simulink model "vehicle_motion_model_final_temp"  (R2021b)
settings: Solver=ode5  StartTime=0.0  StopTime=600  FixedStep=0.001  RelTol=1e-3
StopFcn:
  | % stop simulation callback function
  | figure(1);
  | out.x_gt.data = permute(out.x_gt.data,[3, 1, 2]);
  | plot3(out.x_gt.data(:, 1), out.x_gt.data(:, 2), -out.x_gt.data(:, 3), 'Color', 'r', 'LineWidth', 1.5);
  | legend('Истинная траектория')
  | xlabel('X, \itм');
  | ylabel('Y, \itм');
  | zlabel('Z, \itм');
  | figure(2);
  | plot3(out.x.data(:, 1), out.x.data(:, 2), -out.x.data(:, 3), 'Color', 'b', 'LineWidth', 1.5);
  | hold on;
  | xlabel('X, \itм');
  | ylabel('Y, \itм');
  | zlabel('Z, \itм');
  | % legend('pos')
  | hold on;
  | plot3(out.x_gt.data(:, 1), out.x_gt.data(:, 2), -out.x_gt.data(:, 3), 'Color', 'r', 'LineWidth', 1.5);
  | hold on;
  | legend('Рассчитанная траектория', 'Истинная траектория')
  | % errors
  | figure(3);
  | yyaxis left;
  | plot(out.hor_err_fus.time, out.hor_err_fus.data, 'Color', 'b', 'LineWidth', 1.5);
  | xlabel('время, \itс');
  | ylabel('Горизонтальная ошибка, \itм');
  | hold on;
  | yyaxis right;
  | plot(out.ver_err_fus.time, out.ver_err_fus.data, 'Color', 'r', 'LineWidth', 1.5);
  | ylabel('Вертикальная ошибка, \itм');
  | legend('Горизонтальная позиционная ошибка', 'Вертикальная позиционная ошибка');
  | grid on;
  | figure(4);
  | yyaxis left;
  | plot(out.hor_err_ins.time, out.hor_err_ins.data, '-', 'Color', 'b', 'LineWidth', 1.5);
  | xlabel('время, \itс');
  | ylabel('Горизонтальная ошибка, \itм');
  | hold on;
  | yyaxis right;
  | plot(out.ver_err_ins.time, out.ver_err_ins.data, '-', 'Color', 'r', 'LineWidth', 1.5);
  | ylabel('Вертикальная ошибка, \itм');
  | legend('Горизонтальная позиционная ошибка', 'Вертикальная позиционная ошибка');
  | grid on;
model workspace (MAT data in the model file):
  AxlIxx = 62.3745166667
  AxlM = 160
  Cps = 2
  CzWhlAxl = 557955.087061
  DCT_Param : object (value not decoded)
  Downshift_Speeds = [9.5625 12.9375 16.3125 19.6875 23.0625 26.4375 29.8125 33.1875 36.5625 39.9375 43.3125 46.6875 ... (28 elements, 4x7)]
  F0zWhlAxl = 16132.2380068
  HTCH : object (value not decoded)
  Hmax = 0.25
  KzWhlAxl = 58428920.0848
  NCyl = 6
  Pedal_Positions = [0.1 0.4 0.5 0.9]
  Pstd = 101325
  Q = [1  0  0; 0  1  0; 0  0  1]
  Rair = 287
  SUS : object (value not decoded)
  TRA : object (value not decoded)
  Trans : object (value not decoded)
  Tstd = 293.15
  Upshift_Speeds = [12.9375 16.3125 19.6875 33 26.4375 29.8125 33.1875 52.5 39.9375 43.3125 46.6875 77.25 ... (28 elements, 4x7)]
  VEH : object (value not decoded)
  Vd = 0.00346
  WH : Mass (value not decoded)
  dt3D = 0.05
  f_air = [0 0 0 0 0 0 0 0 0 0 0 0 ... (256 elements, 16x16)]
  f_co = [0 0 0 0 0 0 0 0 0 0 0 0 ... (256 elements, 16x16)]
  f_co2 = [0 0 0 0 0 0 0 0 0 0 0 0 ... (256 elements, 16x16)]
  f_eff = [352.135682859 352.135682859 320.724378192 303.655312657 295.930136708 291.240087194 291.240271258 291.240312459 291.240275452 291.240198499 291.240100781 291.240018769 ... (256 elements, 16x16)]
  f_fuel = [0 0 0 0 0 0 0 0 0 0 0 0 ... (256 elements, 16x16)]
  f_hc = [0 0 0 0 0 0 0 0 0 0 0 0 ... (256 elements, 16x16)]
  f_nox = [0 0 0 0 0 0 0 0 0 0 0 0 ... (256 elements, 16x16)]
  f_pm = [0 0 0 0 0 0 0 0 0 0 0 0 ... (256 elements, 16x16)]
  f_susp_axl_bp = [1 2]
  f_susp_dz_bp = [-0.325022776267 -0.315022776267 -0.305022776267 -0.205022776267 -0.105022776267 -0.00502277626717 0.0949772237328 0.194977223733 0.204977223733 0.214977223733]
  f_susp_dzdot_bp = [-3 -0.3 -0.2 -0.1 0 0.1 0.2 0.3 3]
  f_susp_fmz = [-144070.391448 -93629.24037 -75929.1118915 -20630.5828179 -15385.48216 -10140.3815021 -4895.28084414 349.819813785 -31916.3973792 18437.6709544 -83996.1993354 -33555.0482577 ... (43920 elements, 10x9x61x2x4)]
  f_susp_geom = [0 0 0 0 0 0 0 0 0 0 0 0 ... (3660 elements, 10x61x2x3)]
  f_susp_strgdelta_bp = [-0.523598775598 -0.506145483078 -0.488692190558 -0.471238898038 -0.453785605519 -0.436332312999 -0.418879020479 -0.401425727959 -0.383972435439 -0.366519142919 -0.349065850399 -0.331612557879 ... (61 elements, 1x61)]
  f_tbrake = [0 76.8593923996 105.140482948 131.533638111 157.926793274 176.658631717 176.65727296 176.656856686 176.656879077 176.657093756 176.657404516 176.65772406 ... (256 elements, 16x16)]
  f_tbrake_n_bpt = [0 649.519052838 912.419621844 1175.32019085 1438.22075986 1701.12132886 1964.02189787 2226.92246687 2489.82303588 2752.72360489 3015.62417389 3278.5247429 ... (16 elements, 1x16)]
  f_tbrake_t_bpt = [0 34.6410161514 61.0341713143 87.4273264773 113.82048164 140.213636803 166.606791966 192.999947129 219.393102292 245.786257455 272.179412618 298.572567781 ... (16 elements, 1x16)]
  f_texh = [766.752464599 766.752464599 786.17542386 801.679939032 884.591982581 910.574397722 910.571871054 910.570774534 910.570601632 910.570821151 910.571247242 910.571639815 ... (256 elements, 16x16)]
  f_twc_eff_co = [0.17 0.25 0.45 0.99 0.99 0.99 0.99]
  f_twc_eff_hc = [0.21 0.375 0.75 0.98 0.98 0.98 0.98]
  f_twc_eff_lam = [0.909090909 0.944055944 0.979020979 1 1.013986014 1.048951049 1.083916084]
  f_twc_eff_nox = [0.98 0.98 0.98 0.97 0.05 0.02 0]
  h = 0.134
symbols that are objects in the model workspace (value not decoded): VEH
libraries: aerolibcommonsys x8, sharedtransform x8, sharedutil x7, autolibsharedcommon x7, autolibutils x4, vehdynlibtirecommon x3, dspstat3 x2, mspsensorlib x1, aerolibnav x1, shared6dof x1, autolibshared x1, vehdynlibsuspension x1
(part 2 of 9)

== system vehicle_motion_model_final_temp/Axle Torque ==
  Vehicle : Inport
  1-D Lookup Table : Lookup_n-D  NumberOfTableDimensions=1  BreakpointsForDimension1=[0 3]  Table=[1 0.2]  InternalRulePriority=Speed  RndMeth=Simplest  InputSameDT=on
  1200 Nm Per Rear Wheel : Constant  Value=1200
  Bus Selector : BusSelector  OutputSignals=Vehicle.BdyFrm.Cg.Vel.xdot
  Constant : Constant  Value=0
  Mux : Mux
  Product : Product
  Transfer Fcn : TransferFcn  Denominator=[0.2 1]
  Axle Torque : Outport
  wires:
  Constant/1 -> Mux/2, Mux/1
  1200 Nm Per Rear Wheel/1 -> Product/2
  Transfer Fcn/1 -> Mux/4, Mux/3
  Mux/1 -> Axle Torque/1
  Vehicle/1 -> Bus Selector/1
  Bus Selector/1 -> 1-D Lookup Table/1  "<xdot>"
  Product/1 -> Transfer Fcn/1
  1-D Lookup Table/1 -> Product/1

== system vehicle_motion_model_final_temp/BINS ==
  note: block with biases drift
  note: adis 16384
  note: there will be an assumption for sensor fusion: we consider that IMU acc-ters are identical, so them noises are white, uncorreletad and isotopic (sphere) and therefore mean and covariance matrix are invariant upon rotations (?)
  inputIMU : Inport
  Bus Creator : BusCreator  Inputs=2
  Bus Selector : BusSelector  OutputSignals=Vehicle.BdyFrm.Cg.Abe,Vehicle.BdyFrm.Cg.AngVel,Vehicle.BdyFrm.Cg.AngAcc,Vehicle.BdyFrm.Cg.DCM
  Display : Display
  IMU : mspsensorlib/IMU  Commented=on  DispRefFrame=NED  Temperature=25  MagneticFieldNED=[ 27.5550, -2.4169, -16.0849 ]  MagneticFieldENU=[ -2.4169, 27.5550, 16.0849 ]  SeedDouble=67  SimulateUsing=Interpreted execution  AccelParamsMeasurementRange=Inf  AccelParamsResolution=0  AccelParamsConstantBias=[ 0, 0, 0 ]  AccelParamsAxesMisalignment=[ 100, 0, 0; 0, 100, 0; 0, 0, 100 ]  AccelParamsNoiseDensity=[ 0, 0, 0 ]  AccelParamsBiasInstability=[ 0, 0, 0 ]  AccelParamsRandomWalk=[ 0, 0, 0 ]  AccelParamsTemperatureBias=[ 0, 0, 0 ]  AccelParamsTemperatureScaleFactor=[ 0, 0, 0 ]  GyroParamsMeasurementRange=Inf  GyroParamsResolution=0  GyroParamsConstantBias=[ 0, 0, 0 ]  GyroParamsAxesMisalignment=[ 100, 0, 0; 0, 100, 0; 0, 0, 100 ]  GyroParamsAccelerationBias=[ 0, 0, 0 ]  GyroParamsNoiseDensity=[ 0, 0, 0 ]  GyroParamsBiasInstability=[ 0, 0, 0 ]  GyroParamsRandomWalk=[ 0, 0, 0 ]  GyroParamsTemperatureBias=[ 0, 0, 0 ]  GyroParamsTemperatureScaleFactor=[ 0, 0, 0 ]  MagParamsMeasurementRange=Inf  MagParamsResolution=0  MagParamsConstantBias=[ 0, 0, 0 ]  MagParamsAxesMisalignment=[ 100, 0, 0; 0, 100, 0; 0, 0, 100 ]  MagParamsNoiseDensity=[ 0, 0, 0 ]  MagParamsBiasInstability=[ 0, 0, 0 ]  MagParamsRandomWalk=[ 0, 0, 0 ]  MagParamsTemperatureBias=[ 0, 0, 0 ]  MagParamsTemperatureScaleFactor=[ 0, 0, 0 ]
      settings: SourceProductBaseCode=TF,NV
  Product : Product  Multiplication=Matrix(*)
  RMS : dspstat3/RMS  run=off  directionMode=Each column  dimension=1  reset_popup=None
  RMS1 : dspstat3/RMS  run=off  directionMode=Each column  dimension=1  reset_popup=None
  Scope1 : Scope  NumInputPorts=2
  Scope3 : Scope  NumInputPorts=2
  Subsystem : Subsystem
  Subsystem1 : Subsystem
  Three-axis Inertial Measurement Unit1 : aerolibnav/Three-axis Inertial Measurement Unit  units=Metric (MKS)  imu=[0 0 0]  i_Ts=0  dtype_a=off  w_a=190  z_a=0.707  a_sf_cc=[1 0 0; 0 1 0; 0 0 1]  a_bias=[0, 0, 0]  a_sat="[-inf  -inf  -inf  inf inf inf]"  dtype_g=off  w_g=190  z_g=0.707  g_sf_cc=[1 0 0; 0 1 0; 0 0 1]  g_bias=[0, 0, 0]  g_sens=[0 0 0]  g_sat="[-inf  -inf  -inf  inf inf inf]"  i_rand=on  i_seeds=[23093 23094 23095 23096 23097 23098]  i_pow=[6e-8 6e-8 6e-8 7e-9 7e-9 7e-9]
  Three-axis Inertial Measurement Unit2 : Subsystem  Commented=on  AncestorBlock=aerolibnav/Three-axis Inertial Measurement Unit  mask(Three-axis Inertial Measurement Unit){units=Metric (MKS), imu=[0 0 0], i_Ts=0.001, dtype_a=off, w_a=190, z_a=0.707, a_sf_cc=[1 0 0; 0 1 0; 0 0 1], a_bias=[3e-4,-4e-4, 1e-4], a_sat=[-inf  -inf  -inf  inf inf inf], dtype_g=off, w_g=190, z_g=0.707, g_sf_cc=[1 0 0; 0 1 0; 0 0 1], g_bias=[-2e-4, 4e-4, -1e-4], g_sens=[0 0 0], g_sat=[-inf  -inf  -inf  inf inf inf], i_rand=on, i_seeds=[23093 23094 23095 23096 23097 23098], i_pow=[6e-8 6e-8 6e-8 2e-12 2e-12 2e-12]}
      mask prompts: units "aeroblks:aeroblknav:blockThreeaxisInertialMeasurementUnitParamUnits"; imu "aeroblks:aeroblknav:blockThreeaxisInertialMeasurementUnitParamIMUlocation"; i_Ts "aeroblks:aeroblknav:blockThreeaxisInertialMeasurementUnitParamUpdaterate"; dtype_a "aeroblks:aeroblknav:blockThreeaxisInertialMeasurementUnitParamSecondorderdynamicsforaccelerometer"; w_a "aeroblks:aeroblknav:blockThreeaxisInertialMeasurementUnitParamAccelerometernaturalfrequencyradsec"; z_a "aeroblks:aeroblknav:blockThreeaxisInertialMeasurementUnitParamAccelerometerdampingratio"; a_sf_cc "aeroblks:aeroblknav:blockThreeaxisInertialMeasurementUnitParamAccelerometerscalefactorandcrosscoupling"; a_bias "aeroblks:aeroblknav:blockThreeaxisInertialMeasurementUnitParamAccelerometermeasurementbias"; a_sat "aeroblks:aeroblknav:blockThreeaxisInertialMeasurementUnitParamAccelerometerupperandlowerlimits"; dtype_g "aeroblks:aeroblknav:blockThreeaxisInertialMeasurementUnitParamSecondorderdynamicsforgyro"; w_g "aeroblks:aeroblknav:blockThreeaxisInertialMeasurementUnitParamGyronaturalfrequencyradsec"; z_g "aeroblks:aeroblknav:blockThreeaxisInertialMeasurementUnitParamGyrodampingratio"; g_sf_cc "aeroblks:aeroblknav:blockThreeaxisInertialMeasurementUnitParamGyroscalefactorsandcrosscoupling"; g_bias "aeroblks:aeroblknav:blockThreeaxisInertialMeasurementUnitParamGyromeasurementbias"; g_sens "aeroblks:aeroblknav:blockThreeaxisInertialMeasurementUnitParamGsensitivebias"; g_sat "aeroblks:aeroblknav:blockThreeaxisInertialMeasurementUnitParamGyroupperandlowerlimits"; i_rand "aeroblks:aeroblknav:blockThreeaxisInertialMeasurementUnitParamNoiseon"; i_seeds "aeroblks:aeroblknav:blockThreeaxisInertialMeasurementUnitParamNoiseseeds"; i_pow "aeroblks:aeroblknav:blockThreeaxisInertialMeasurementUnitParamNoisepower"
      mask help: aeroblks:aeroblknav:blockThreeaxisInertialMeasurementUnitDesc
      mask init:
      | block = gcb;   
      | ports=aeroicon('aeroblkimu','icon');
      mask Help: eval('asbhelp');
      mask TypeOptions units: aeroblks:aeroblknav:blockThreeaxisInertialMeasurementUnitParamComboMetricMKS | aeroblks:aeroblknav:blockThreeaxisInertialMeasurementUnitParamComboEnglish
      mask Callback dtype_a: aeroicon('aeroblkimu')
      mask Callback dtype_g: aeroicon('aeroblkimu')
      mask Callback i_rand: aeroicon('aeroblkimu')
      mask DialogControl ParameterTabVar0 Prompt: Main
      mask DialogControl units Prompt: Units:
      mask DialogControl imu Prompt: IMU location:
      mask DialogControl i_Ts Prompt: Update rate:
      mask DialogControl ParameterTabVar01 Prompt: Accelerometer
      mask DialogControl dtype_a Prompt: Second-order dynamics for accelerometer
      mask DialogControl w_a Prompt: Accelerometer natural frequency (rad/sec):
      mask DialogControl z_a Prompt: Accelerometer damping ratio:
      mask DialogControl a_sf_cc Prompt: Accelerometer scale factor and cross-coupling:
      mask DialogControl a_bias Prompt: Accelerometer measurement bias:
      mask DialogControl a_sat Prompt: Accelerometer upper and lower limits:
      mask DialogControl ParameterTabVar012 Prompt: Gyroscope
      mask DialogControl dtype_g Prompt: Second-order dynamics for gyro
      mask DialogControl w_g Prompt: Gyro natural frequency (rad/sec):
      mask DialogControl z_g Prompt: Gyro damping ratio:
      mask DialogControl g_sf_cc Prompt: Gyro scale factors and cross-coupling:
      mask DialogControl g_bias Prompt: Gyro measurement bias:
      mask DialogControl g_sens Prompt: G-sensitive bias:
      mask DialogControl g_sat Prompt: Gyro upper and lower limits:
      mask DialogControl ParameterTabVar0123 Prompt: Noise
      mask DialogControl i_rand Prompt: Noise on
      mask DialogControl i_seeds Prompt: Noise seeds:
      mask DialogControl i_pow Prompt: Noise power:
      mask Display:
      | port_label(ports(1).type,ports(1).port,ports(1).txt,'texmode','on');
      | port_label(ports(2).type,ports(2).port,ports(2).txt,'texmode','on');
      | port_label(ports(3).type,ports(3).port,ports(3).txt,'texmode','on');
      | port_label(ports(4).type,ports(4).port,ports(4).txt,'texmode','on');
      | port_label(ports(5).type,ports(5).port,ports(5).txt,'texmode','on');
      | port_label(ports(6).type,ports(6).port,ports(6).txt,'texmode','on');
      | port_label(ports(7).type,ports(7).port,ports(7).txt,'texmode','on');
  Three-axis Inertial Measurement Unit4 : Subsystem  Commented=on  AncestorBlock=aerolibnav/Three-axis Inertial Measurement Unit  mask(Three-axis Inertial Measurement Unit){units=Metric (MKS), imu=[0 0 0], i_Ts=0.01, dtype_a=off, w_a=190, z_a=0.707, a_sf_cc=[1 0 0; 0 1 0; 0 0 1], a_bias=[3e-4,-4e-4, 1e-4], a_sat=[-inf  -inf  -inf  inf inf inf], dtype_g=off, w_g=190, z_g=0.707, g_sf_cc=[1 0 0; 0 1 0; 0 0 1], g_bias=[-2e-4, 4e-4, -1e-4], g_sens=[0 0 0], g_sat=[-inf  -inf  -inf  inf inf inf], i_rand=on, i_seeds=[23093 23094 23095 23096 23097 23098], i_pow=[7e-9 7e-9 7e-9 6e-8 6e-8 6e-8]}
      mask prompts: units "aeroblks:aeroblknav:blockThreeaxisInertialMeasurementUnitParamUnits"; imu "aeroblks:aeroblknav:blockThreeaxisInertialMeasurementUnitParamIMUlocation"; i_Ts "aeroblks:aeroblknav:blockThreeaxisInertialMeasurementUnitParamUpdaterate"; dtype_a "aeroblks:aeroblknav:blockThreeaxisInertialMeasurementUnitParamSecondorderdynamicsforaccelerometer"; w_a "aeroblks:aeroblknav:blockThreeaxisInertialMeasurementUnitParamAccelerometernaturalfrequencyradsec"; z_a "aeroblks:aeroblknav:blockThreeaxisInertialMeasurementUnitParamAccelerometerdampingratio"; a_sf_cc "aeroblks:aeroblknav:blockThreeaxisInertialMeasurementUnitParamAccelerometerscalefactorandcrosscoupling"; a_bias "aeroblks:aeroblknav:blockThreeaxisInertialMeasurementUnitParamAccelerometermeasurementbias"; a_sat "aeroblks:aeroblknav:blockThreeaxisInertialMeasurementUnitParamAccelerometerupperandlowerlimits"; dtype_g "aeroblks:aeroblknav:blockThreeaxisInertialMeasurementUnitParamSecondorderdynamicsforgyro"; w_g "aeroblks:aeroblknav:blockThreeaxisInertialMeasurementUnitParamGyronaturalfrequencyradsec"; z_g "aeroblks:aeroblknav:blockThreeaxisInertialMeasurementUnitParamGyrodampingratio"; g_sf_cc "aeroblks:aeroblknav:blockThreeaxisInertialMeasurementUnitParamGyroscalefactorsandcrosscoupling"; g_bias "aeroblks:aeroblknav:blockThreeaxisInertialMeasurementUnitParamGyromeasurementbias"; g_sens "aeroblks:aeroblknav:blockThreeaxisInertialMeasurementUnitParamGsensitivebias"; g_sat "aeroblks:aeroblknav:blockThreeaxisInertialMeasurementUnitParamGyroupperandlowerlimits"; i_rand "aeroblks:aeroblknav:blockThreeaxisInertialMeasurementUnitParamNoiseon"; i_seeds "aeroblks:aeroblknav:blockThreeaxisInertialMeasurementUnitParamNoiseseeds"; i_pow "aeroblks:aeroblknav:blockThreeaxisInertialMeasurementUnitParamNoisepower"
      mask help: aeroblks:aeroblknav:blockThreeaxisInertialMeasurementUnitDesc
      mask init:
      | block = gcb;   
      | ports=aeroicon('aeroblkimu','icon');
      mask Help: eval('asbhelp');
      mask TypeOptions units: aeroblks:aeroblknav:blockThreeaxisInertialMeasurementUnitParamComboMetricMKS | aeroblks:aeroblknav:blockThreeaxisInertialMeasurementUnitParamComboEnglish
      mask Callback dtype_a: aeroicon('aeroblkimu')
      mask Callback dtype_g: aeroicon('aeroblkimu')
      mask Callback i_rand: aeroicon('aeroblkimu')
      mask DialogControl ParameterTabVar0 Prompt: Main
      mask DialogControl units Prompt: Units:
      mask DialogControl imu Prompt: IMU location:
      mask DialogControl i_Ts Prompt: Update rate:
      mask DialogControl ParameterTabVar01 Prompt: Accelerometer
      mask DialogControl dtype_a Prompt: Second-order dynamics for accelerometer
      mask DialogControl w_a Prompt: Accelerometer natural frequency (rad/sec):
      mask DialogControl z_a Prompt: Accelerometer damping ratio:
      mask DialogControl a_sf_cc Prompt: Accelerometer scale factor and cross-coupling:
      mask DialogControl a_bias Prompt: Accelerometer measurement bias:
      mask DialogControl a_sat Prompt: Accelerometer upper and lower limits:
      mask DialogControl ParameterTabVar012 Prompt: Gyroscope
      mask DialogControl dtype_g Prompt: Second-order dynamics for gyro
      mask DialogControl w_g Prompt: Gyro natural frequency (rad/sec):
      mask DialogControl z_g Prompt: Gyro damping ratio:
      mask DialogControl g_sf_cc Prompt: Gyro scale factors and cross-coupling:
      mask DialogControl g_bias Prompt: Gyro measurement bias:
      mask DialogControl g_sens Prompt: G-sensitive bias:
      mask DialogControl g_sat Prompt: Gyro upper and lower limits:
      mask DialogControl ParameterTabVar0123 Prompt: Noise
      mask DialogControl i_rand Prompt: Noise on
      mask DialogControl i_seeds Prompt: Noise seeds:
      mask DialogControl i_pow Prompt: Noise power:
      mask Display:
      | port_label(ports(1).type,ports(1).port,ports(1).txt,'texmode','on');
      | port_label(ports(2).type,ports(2).port,ports(2).txt,'texmode','on');
      | port_label(ports(3).type,ports(3).port,ports(3).txt,'texmode','on');
      | port_label(ports(4).type,ports(4).port,ports(4).txt,'texmode','on');
      | port_label(ports(5).type,ports(5).port,ports(5).txt,'texmode','on');
      | port_label(ports(6).type,ports(6).port,ports(6).txt,'texmode','on');
      | port_label(ports(7).type,ports(7).port,ports(7).txt,'texmode','on');
  center of gravity : Constant  Value=[0;0;0]
  gravity vector : Constant  Value=[0;0;9.8]  VectorParams1D=off
  BINSOut : Outport
  tag scope: g=global
  wires:
  gravity vector/1 -> [g], Product/2  "g"
  center of gravity/1 -> Three-axis Inertial Measurement Unit1/4
  inputIMU/1 -> Bus Selector/1
  Bus Selector/1 -> Three-axis Inertial Measurement Unit1/1, Subsystem/1(True)  "<Abe>"
  Bus Selector/2 -> Three-axis Inertial Measurement Unit1/2, Subsystem1/1(True)  "<AngVel>"
  Bus Selector/3 -> Three-axis Inertial Measurement Unit1/3  "<AngAcc>"
  Three-axis Inertial Measurement Unit1/2 -> Subsystem1/2(BINS), RMS/1, Scope3/2, Bus Creator/2  "Wmeas"
  Three-axis Inertial Measurement Unit1/1 -> Subsystem/2(BINS), Scope3/1, RMS1/1, Bus Creator/1  "Ameas"
  Bus Creator/1 -> Display/1, BINSOut/1
  RMS/1 -> Scope1/2
  RMS1/1 -> Scope1/1
  Product/1 -> Three-axis Inertial Measurement Unit1/5
  Bus Selector/4 -> Product/1  "<DCM>"

== system vehicle_motion_model_final_temp/BINS kinematics Euler ==
  BINSout : Inport
  Bus Creator : BusCreator  Inputs=3
  Bus Selector : BusSelector  OutputSignals=Wmeas,Ameas
  Bus Selector1 : BusSelector  OutputSignals=Ang,Vel,Disp
  Derivative : Derivative
  Divide1 : Product  Inputs=/*  Multiplication=Matrix(*)
  Integrator : Integrator  InitialConditionSource=external
  Integrator1 : Integrator  InitialConditionSource=external
  Integrator2 : Integrator  InitialConditionSource=external
  Subsystem : Subsystem
  Subsystem1 : Subsystem
  Sum : Sum  Inputs=++|
  Turning equations : MATLAB Function  TreatAsAtomicUnit=on
  calc rotation matrix : MATLAB Function  TreatAsAtomicUnit=on
  gravity vector : Constant  Value=[0;0;9.8]  VectorParams1D=off
  EulerOut : Outport
  wires:
  Turning equations/1(dv_dt) -> Integrator/1
  Integrator/1 -> Bus Creator/1, calc rotation matrix/1(ang), Subsystem1/2(BINS), Turning equations/1(ang)  "CalcAng"
  Bus Selector1/2 -> Integrator1/2  "<Vel>"
  Integrator1/1 -> Bus Creator/2, Integrator2/1  "CalcVel"
  BINSout/1 -> Bus Selector/1
  calc rotation matrix/1(DCM_calc) -> Divide1/1
  Divide1/1 -> Sum/2
  gravity vector/1 -> Sum/1
  Bus Creator/1 -> EulerOut/1
  Sum/1 -> Subsystem/1(True), Integrator1/1
  Derivative/1 -> Subsystem/2(BINS)
  Bus Selector/2 -> Divide1/2  "<Ameas>"
  Bus Selector/1 -> Turning equations/2(w)  "<Wmeas>"
  [InertFrmCg] -> Bus Selector1/1
  Integrator2/1 -> Bus Creator/3  "CalcPos"
  Bus Selector1/1 -> Integrator/2  "<Ang>"
  Bus Selector1/3 -> Integrator2/2  "<Disp>"
  [InertFrmAng] -> Subsystem1/1(True)
  [InertFrmVel] -> Derivative/1

== system vehicle_motion_model_final_temp/BINS kinematics quaternion ==
  BINSout : Inport
  Bus Creator : BusCreator  Inputs=3
  Bus Selector : BusSelector  OutputSignals=Wmeas,Ameas
  Bus Selector1 : BusSelector  OutputSignals=Ang,Vel,Disp
  DCM calc : MATLAB Function  TreatAsAtomicUnit=on
  Divide1 : Product  Inputs=/*  Multiplication=Matrix(*)
  Integrator : Integrator  InitialConditionSource=external
  Integrator1 : Integrator  InitialConditionSource=external
  Integrator2 : Integrator  InitialConditionSource=external
  Manual Switch2 : ManualSwitch  CurrentSetting=0
  Manual Switch3 : ManualSwitch
  Manual Switch4 : ManualSwitch  CurrentSetting=0
  Quaternions to Direction Cosine Matrix : sharedtransform/Quaternions to  Direction Cosine Matrix  aMode=aMode
      settings: SourceProductBaseCode=AE,PW,DR,MT,UV,VE
  Quaternions to Rotation Angles : sharedtransform/Quaternions to Rotation Angles  rotationOrder=ZYX  aMode=aMode
      settings: SourceProductBaseCode=AE,PW,DR,MT,UV,VE
  Rotation Angles to Quaternions1 : sharedtransform/Rotation Angles to Quaternions  rotationOrder=ZYX  aMode=aMode
      settings: SourceProductBaseCode=AE,PW,DR,MT,UV,VE
  Selector : Selector  InputPortWidth=3  IndexOptions=Index vector (dialog)  Indices=[3 2 1]  OutputSizes=1
  Selector1 : Selector  InputPortWidth=3  IndexOptions=Index vector (dialog)  Indices=[3 2 1]  OutputSizes=1
  Sum : Sum  Inputs=|++
  To angles : MATLAB Function  TreatAsAtomicUnit=on
  Turning equations : MATLAB Function  TreatAsAtomicUnit=on
  calc begin values quater : MATLAB Function  TreatAsAtomicUnit=on
  gravity vector : Constant  Value=[0;0;10]
  QuatOut : Outport
  wires:
  Integrator1/1 -> Bus Creator/2, Integrator2/1  "CalcVel"
  gravity vector/1 -> Sum/1
  Sum/1 -> Integrator1/1
  Turning equations/1(dl_dt) -> Integrator/1
  Manual Switch2/1 -> Integrator/2
  Integrator/1 -> DCM calc/1(q), Quaternions to Direction Cosine Matrix/1, To angles/1(q), Quaternions to Rotation Angles/1, Turning equations/1(quat)
  Divide1/1 -> Sum/2
  Bus Creator/1 -> QuatOut/1
  Selector1/1 -> Rotation Angles to Quaternions1/1
  Quaternions to Direction Cosine Matrix/1 -> Manual Switch3/2
  Bus Selector/2 -> Divide1/2  "<Ameas>"
  Quaternions to Rotation Angles/1 -> Selector/1
  calc begin values quater/1(l) -> Manual Switch2/2
  Rotation Angles to Quaternions1/1 -> Manual Switch2/1
  DCM calc/1(DCM_calc) -> Manual Switch3/1
  Manual Switch3/1 -> Divide1/1
  To angles/1(ang) -> Manual Switch4/1
  Selector/1 -> Manual Switch4/2
  Manual Switch4/1 -> Bus Creator/1  "CalcAng"
  Integrator2/1 -> Bus Creator/3  "CalcPos"
  [InertFrmCg] -> Bus Selector1/1
  Bus Selector1/1 -> calc begin values quater/1(ang), Selector1/1  "<Ang>"
  Bus Selector1/2 -> Integrator1/2  "<Vel>"
  Bus Selector1/3 -> Integrator2/2  "<Disp>"
  BINSout/1 -> Bus Selector/1
  Bus Selector/1 -> Turning equations/2(w)  "<Wmeas>"

== system vehicle_motion_model_final_temp/Calc errors ==
  note: vel
  note: pos
  note: ang
  calc : Inport
  Bus Selector : BusSelector  OutputSignals=Disp,Vel,Ang
  Bus Selector1 : BusSelector  OutputSignals=CalcPos,CalcVel,CalcAng
  Scope1 : Scope  NumInputPorts=3
  Scope2 : Scope  NumInputPorts=3
  Scope3 : Scope  NumInputPorts=2
  Scope4 : Scope  NumInputPorts=3
  Subsystem : Subsystem
  Sum1 : Sum  Inputs=+-|
  Sum2 : Sum  Inputs=+-|
  Sum3 : Sum  Inputs=+-|
  wires:
  Bus Selector1/3 -> Scope2/2, Sum3/2  "<CalcAng>"
  Sum3/1 -> Scope2/3
  Bus Selector/1 -> Subsystem/1(<Disp>), Sum2/1, Scope4/1  "<Disp>"
  Bus Selector1/1 -> Subsystem/2(<CalcPos>), Scope4/2, Sum2/2  "<CalcPos>"
  Bus Selector/2 -> Scope1/1, Sum1/1  "<Vel>"
  [InertFrmCg] -> Bus Selector/1
  Sum2/1 -> Scope4/3
  Bus Selector/3 -> Scope2/1, Sum3/1  "<Ang>"
  Bus Selector1/2 -> Scope1/2, Sum1/2  "<CalcVel>"
  Sum1/1 -> Scope1/3
  calc/1 -> Bus Selector1/1
  Subsystem/1(HorError) -> Scope3/1
  Subsystem/2(VertError) -> Scope3/2

== system vehicle_motion_model_final_temp/Calc errors1 ==
  note: pos
  note: ang
  note: vel
  calc : Inport
  Bus Selector2 : BusSelector  OutputSignals=Disp,Vel,Ang
  Bus Selector3 : BusSelector  OutputSignals=CalcPos,CalcVel,CalcAng
  Scope1 : Scope  NumInputPorts=2
  Scope2 : Scope  NumInputPorts=3
  Scope3 : Scope  NumInputPorts=3
  Scope4 : Scope  NumInputPorts=3
  Subsystem1 : Subsystem
  Sum4 : Sum  Inputs=+-|
  Sum5 : Sum  Inputs=+-|
  Sum6 : Sum  Inputs=+-|
  wires:
  Sum5/1 -> Scope4/3
  Bus Selector3/1 -> Subsystem1/2(<CalcPos>), Scope4/2, Sum5/2  "<CalcPos>"
  Bus Selector3/3 -> Scope3/2, Sum6/2  "<CalcAng>"
  Bus Selector2/3 -> Scope3/1, Sum6/1  "<Ang>"
  Bus Selector3/2 -> Scope2/2, Sum4/2  "<CalcVel>"
  [InertFrmCg] -> Bus Selector2/1
  Bus Selector2/1 -> Subsystem1/1(<Disp>), Scope4/1, Sum5/1  "<Disp>"
  Bus Selector2/2 -> Scope2/1, Sum4/1  "<Vel>"
  Sum4/1 -> Scope2/3
  calc/1 -> Bus Selector3/1
  Sum6/1 -> Scope3/3
  Subsystem1/2(VertError) -> Scope1/2
  Subsystem1/1(HorError) -> Scope1/1

== system vehicle_motion_model_final_temp/Calc errors2 ==
  note: ab, wb, g
  note: ang
  note: vel
  note: pos
  calc : Inport
  Bus Selector : BusSelector  OutputSignals=Disp,Vel,Ang
  Scope4 : Scope  NumInputPorts=2
  Scope{5..8} (4 alike) : Scope  NumInputPorts=3
  Selector : Selector  InputPortWidth=19  IndexOptions=Index vector (dialog)  Indices=[1 2 3]  OutputSizes=1
  Selector1 : Selector  InputPortWidth=19  IndexOptions=Index vector (dialog)  Indices=[4 5 6]  OutputSizes=1
  Selector2 : Selector  InputPortWidth=19  IndexOptions=Index vector (dialog)  Indices=[7 8 9 10]  OutputSizes=1
  Selector3 : Selector  InputPortWidth=19  IndexOptions=Index vector (dialog)  Indices=[11 12 13]  OutputSizes=1
  Selector4 : Selector  InputPortWidth=19  IndexOptions=Index vector (dialog)  Indices=[14 15 16]  OutputSizes=1
  Selector5 : Selector  InputPortWidth=19  IndexOptions=Index vector (dialog)  Indices=[17 18 19]  OutputSizes=1
  Subsystem : Subsystem
  Sum1 : Sum  Inputs=+-|
  Sum2 : Sum  Inputs=+-|
  Sum3 : Sum  Inputs=+-|
  To Workspace1 : ToWorkspace  VariableName=hor_err_fus  SaveFormat=Timeseries  SampleTime=-1
  To Workspace2 : ToWorkspace  VariableName=ver_err_fus  SaveFormat=Timeseries  SampleTime=-1
  To angles : MATLAB Function  TreatAsAtomicUnit=on
  wires:
  calc/1 -> Selector2/1, Selector3/1, Selector4/1, Selector5/1, Selector1/1, Selector/1
  Sum1/1 -> Scope8/3
  Bus Selector/2 -> Scope8/1, Sum1/1  "<Vel>"
  Selector1/1 -> Scope8/2, Sum1/2
  Sum3/1 -> Scope7/3
  Bus Selector/3 -> Scope7/1, Sum3/1  "<Ang>"
  Sum2/1 -> Scope6/3
  Selector3/1 -> Scope5/1
  Selector4/1 -> Scope5/2
  Selector5/1 -> Scope5/3
  Selector2/1 -> To angles/1(qat)
  To angles/1(ang) -> Scope7/2, Sum3/2
  [InertFrmCg] -> Bus Selector/1
  Bus Selector/1 -> Subsystem/1(<Disp>), Scope6/1, Sum2/1  "<Disp>"
  Selector/1 -> Subsystem/2(<CalcPos>), Scope6/2, Sum2/2
  Subsystem/1(HorError) -> To Workspace1/1, Scope4/1
  Subsystem/2(VertError) -> To Workspace2/1, Scope4/2

== system vehicle_motion_model_final_temp/Calc errors3 ==
  note: ab, wb, g
  note: ang
  note: vel
  note: pos
  calc : Inport
  Bus Selector : BusSelector  OutputSignals=Disp,Vel,Ang
  Scope{1..3,5} (4 alike) : Scope  NumInputPorts=3
  Scope4 : Scope  NumInputPorts=2
  Selector : Selector  InputPortWidth=19  IndexOptions=Index vector (dialog)  Indices=[1 2 3]  OutputSizes=1
  Selector1 : Selector  InputPortWidth=19  IndexOptions=Index vector (dialog)  Indices=[4 5 6]  OutputSizes=1
  Selector2 : Selector  InputPortWidth=19  IndexOptions=Index vector (dialog)  Indices=[7 8 9 10]  OutputSizes=1
  Selector3 : Selector  InputPortWidth=19  IndexOptions=Index vector (dialog)  Indices=[11 12 13]  OutputSizes=1
  Selector4 : Selector  InputPortWidth=19  IndexOptions=Index vector (dialog)  Indices=[14 15 16]  OutputSizes=1
  Selector5 : Selector  InputPortWidth=19  IndexOptions=Index vector (dialog)  Indices=[17 18 19]  OutputSizes=1
  Subsystem : Subsystem
  Sum1 : Sum  Inputs=+-|
  Sum2 : Sum  Inputs=+-|
  Sum3 : Sum  Inputs=+-|
  To Workspace1 : ToWorkspace  VariableName=hor_err_ins  SaveFormat=Timeseries  SampleTime=-1
  To Workspace2 : ToWorkspace  VariableName=ver_err_ins  SaveFormat=Timeseries  SampleTime=-1
  To angles : MATLAB Function  TreatAsAtomicUnit=on
  wires:
  calc/1 -> Selector2/1, Selector3/1, Selector4/1, Selector5/1, Selector1/1, Selector/1
  Sum1/1 -> Scope1/3
  Bus Selector/2 -> Scope1/1, Sum1/1  "<Vel>"
  Selector1/1 -> Scope1/2, Sum1/2
  Sum3/1 -> Scope2/3
  Bus Selector/3 -> Scope2/1, Sum3/1  "<Ang>"
  Sum2/1 -> Scope5/3
  Selector3/1 -> Scope3/1
  Selector4/1 -> Scope3/2
  Selector5/1 -> Scope3/3
  Selector2/1 -> To angles/1(qat)
  To angles/1(ang) -> Scope2/2, Sum3/2
  [InertFrmCg] -> Bus Selector/1
  Bus Selector/1 -> Subsystem/1(<Disp>), Scope5/1, Sum2/1  "<Disp>"
  Selector/1 -> Subsystem/2(<CalcPos>), Scope5/2, Sum2/2
  Subsystem/1(HorError) -> To Workspace1/1, Scope4/1
  Subsystem/2(VertError) -> To Workspace2/1, Scope4/2

== system vehicle_motion_model_final_temp/Odometer ==
  note: for wheel radius check
  Wheels : Inport
  Bus Selector1 : BusSelector  OutputSignals=TireFrame.Omega
  Constant : Constant  Value=0.50673
  Demux : Demux
  Demux1 : Demux
  Divide : Product  Inputs=/*
  Mux : Mux
  Radius : Gain  Gain=0.50673
  Random Number : RandomNumber  Variance=1e-4  Seed=52352346346  SampleTime=0.1
  Random Number1 : RandomNumber  Variance=1e-4  Seed=234234  SampleTime=0.1
  Random Number2 : RandomNumber  Variance=0.0001  Seed=2131231  SampleTime=0.1
  Random Number3 : RandomNumber  Variance=0.0001  Seed=342342  SampleTime=0.1
  Scope1 : Scope
  Scope2 : Scope
  Scope4 : Scope  NumInputPorts=3
  Scope6 : Scope
  Selector : Selector  InputPortWidth=4  IndexOptions=Index vector (dialog)  Indices=[3 4]  OutputSizes=1
  Sum{1..4} (4 alike) : Sum
  Sum5 : Sum  Inputs=+-
  Sum6 : Sum  Inputs=+-|
  WhlVel : Outport
  wires:
  Bus Selector1/1 -> Radius/1  "<Omega>"
  Wheels/1 -> Bus Selector1/1
  Random Number/1 -> Sum2/2
  Radius/1 -> Demux/1
  Demux/4 -> Sum5/2, Sum2/1
  Random Number1/1 -> Sum1/2
  Demux/2 -> Sum3/1
  Random Number2/1 -> Sum3/2
  Demux/1 -> Sum4/1
  Demux/3 -> Sum1/1
  Random Number3/1 -> Sum4/2
  Sum4/1 -> Mux/1
  Sum2/1 -> Mux/4
  Sum1/1 -> Mux/3
  Sum3/1 -> Mux/2
  Mux/1 -> Scope6/1, WhlVel/1
  [WhlVx] -> Demux1/1
  Divide/1 -> Scope1/1
  Demux1/4 -> Divide/1, Sum5/1
  Sum5/1 -> Divide/2
  Sum6/1 -> Scope2/1, Scope4/3
  Constant/1 -> Scope4/2, Sum6/2
  [Re] -> Selector/1
  Selector/1 -> Scope4/1, Sum6/1

== system vehicle_motion_model_final_temp/Odometer kinimatics ==
  WhlVel : Inport
  Orientation : Inport  Port=2
  BINSout : Inport  Port=3
  Demux : Demux  Outputs=2
  Divide1 : Product  Inputs=/*  Multiplication=Matrix(*)
  From : From  Commented=on  GotoTag=InertFrmAng  TagVisibility=global
  From1 : From  Commented=on  GotoTag=InertFrmPos  TagVisibility=global
  From2 : From  Commented=on  GotoTag=BdyFrmAngVel  TagVisibility=global
  MATLAB Function1 : MATLAB Function  TreatAsAtomicUnit=on
  Quaternions to Direction Cosine Matrix : sharedtransform/Quaternions to  Direction Cosine Matrix  aMode=aMode
      settings: SourceProductBaseCode=AE,PW,DR,MT,UV,VE
  Scope1 : Scope
  Scope2 : Scope  NumInputPorts=3
  Scope4 : Scope
  Scope6 : Scope  NumInputPorts=3
  Selector2 : Selector  InputPortWidth=19  IndexOptions=Index vector (dialog)  Indices=[7 8 9 10]  OutputSizes=1
  Sum : Sum  Inputs=-+
  Sum1 : Sum  Inputs=-+
  Terminator : Terminator
  VEH.RearAxlePositionfromCG : Constant  Value=VEH.RearAxlePositionfromCG
  VEH.TrackWidth : Constant  Value=VEH.TrackWidth
  InertFrmOdoVel : Outport
  wires:
  VEH.TrackWidth/1 -> MATLAB Function1/5(T_r)
  From1/1 -> MATLAB Function1/2(InertFrmPos)
  MATLAB Function1/1(v_eb) -> Divide1/2, Scope2/1, Sum/1
  VEH.RearAxlePositionfromCG/1 -> MATLAB Function1/6(l_br)
  Sum/1 -> Scope4/1, Scope2/3
  [BdyFrmVel] -> Scope2/2, Sum/2
  From/1 -> MATLAB Function1/3(InertFrmAng)
  BINSout/1 -> Demux/1
  Demux/1 -> Terminator/1
  Demux/2 -> MATLAB Function1/4(omega_eb)
  Quaternions to Direction Cosine Matrix/1 -> Divide1/1
  Divide1/1 -> Scope6/2, Sum1/1, InertFrmOdoVel/1
  Sum1/1 -> Scope1/1, Scope6/3
  [InertFrmVel] -> Scope6/1, Sum1/2
  Orientation/1 -> Selector2/1
  Selector2/1 -> Quaternions to Direction Cosine Matrix/1
  WhlVel/1 -> MATLAB Function1/1(WhlVel)

== system vehicle_motion_model_final_temp/Prediction step (BINS) ==
  BINSout : Inport
  Constant9 : Constant  Value=0
  Delay13 : Delay  DelayLength=1  InitialConditionSource=Input port  InitialCondition=0
      settings: InputPortMap=u0,p4
  Delay14 : Delay  DelayLength=1  InitialConditionSource=Input port  InitialCondition=0
      settings: InputPortMap=u0,p4
  Initial State : Subsystem
  Prediction : MATLAB Function  TreatAsAtomicUnit=on
  Subsystem4 : Subsystem
  x : Outport
  wires:
  Initial State/1(Out1) -> Delay13/2
  Delay14/1 -> Prediction/2(P_)
  Delay13/1 -> Prediction/1(x_)
  Constant9/1 -> Delay14/2
  Subsystem4/1(dT) -> Prediction/3(dT)
  BINSout/1 -> Prediction/4(BINS_output)
  Prediction/2(P) -> Delay14/1
  Prediction/1(x) -> x/1, Delay13/1

== system vehicle_motion_model_final_temp/Sensor fusion ==
  BINSout : Inport
  z : Inport  Port=2
  Clock1 : Clock
  Constant9 : Constant  Value=0
  Correction : MATLAB Function  TreatAsAtomicUnit=on
  Delay12 : Delay  DelayLength=1  InitialCondition=0
  Delay13 : Delay  DelayLength=1  InitialConditionSource=Input port  InitialCondition=0
      settings: InputPortMap=u0,p4
  Delay14 : Delay  DelayLength=1  InitialConditionSource=Input port  InitialCondition=0
      settings: InputPortMap=u0,p4
  Initial State : Subsystem
  Prediction : MATLAB Function  TreatAsAtomicUnit=on
  Subsystem4 : Subsystem
  To Workspace1 : ToWorkspace  VariableName=x  SaveFormat=Timeseries  SampleTime=-1
  x : Outport
  wires:
  z/1 -> Correction/4(z)
  Initial State/1(Out1) -> Delay13/2
  BINSout/1 -> Delay12/1
  Delay14/1 -> Prediction/2(P_)
  Delay13/1 -> Prediction/1(x_)
  Constant9/1 -> Delay14/2
  Subsystem4/1(dT) -> Prediction/3(dT)
  Delay12/1 -> Prediction/4(BINS_output)
  Correction/2(P) -> Delay14/1
  Correction/1(x) -> To Workspace1/1, Delay13/1
  Prediction/1(x) -> x/1, Correction/1("x ")
  Prediction/2(P) -> Correction/2("P ")
  Clock1/1 -> Correction/3(T)

== system vehicle_motion_model_final_temp/Sine Steer ==
  Clock : Clock
  Constant1 : Constant  Value=0
  Gain : Gain  Gain=2*pi/30
  Gain1 : Gain  Gain=0
  Gain2 : Gain  Gain=pi/10
  Mux : Mux
  Sin : Trigonometry
  Steer : Outport
  wires:
  Mux/1 -> Steer/1
  Clock/1 -> Gain/1
  Sin/1 -> Gain2/1
  Gain/1 -> Sin/1
  Gain2/1 -> Mux/1, Mux/2
  Constant1/1 -> Mux/4, Mux/3

== system vehicle_motion_model_final_temp/Two-Axle Vehicle ==
  Steering : Inport
  Axle Torque : Inport  Port=2
  Brake Press : Inport  Port=3
  Ground Input : Inport  Port=4
  Bus Creator : BusCreator  Inputs=2
  Bus Selector : BusSelector  OutputSignals=z,mu
  Vehicle Body : Subsystem  Variant=on  VariantControlMode=label  LabelModeActiveChoice=1
  Vehicle Suspension : Subsystem
      mask Display: image('suspsacoil.png')
  Wheels and Tires : Subsystem
      mask Display: image('wheel3dof.png')
  Vehicle : Outport
  Wheels : Outport  Port=2
  wires:
  Bus Selector/1 -> Wheels and Tires/4(Ground Input)  "<z>"
  Vehicle Suspension/1(Suspension) -> Bus Creator/2, Vehicle Body/1(Suspension), Wheels and Tires/1(Suspension)  "Suspension"
  Vehicle Body/1(Vehicle) -> Bus Creator/1, Vehicle Suspension/3(Vehicle)  "Vehicle"
  Wheels and Tires/1(Wheels) -> Wheels/1, Vehicle Suspension/2(Wheels)  "Wheels"
  Bus Selector/2 -> Wheels and Tires/5(Friction)  "<mu>"
  Axle Torque/1 -> Wheels and Tires/2(Axle Torque)
  Steering/1 -> Vehicle Suspension/1(Steering)
  Brake Press/1 -> Wheels and Tires/3(Brake Press)
  Ground Input/1 -> Bus Selector/1
  Bus Creator/1 -> Vehicle/1

== system vehicle_motion_model_final_temp/Vehicle Ground Input ==
  Bus Creator : BusCreator  Inputs=4
  Bus Creator2 : BusCreator  Inputs=4
  Bus Creator3 : BusCreator  Inputs=2
  Constant1 : Constant  Value=zeros(4,1)
  Demux : Demux
  Demux1 : Demux
  Friction : Constant  Value=ones(4,1).*1.0
  Signal Specification : SignalSpecification  Unit=m
  Signal Specification1 : SignalSpecification  Unit=1
  Ground : Outport  VectorParamsAs1DForOutWhenUnconnected=off
  wires:
  Bus Creator3/1 -> Ground/1
  Signal Specification1/1 -> Demux1/1
  Friction/1 -> Signal Specification1/1
  Bus Creator2/1 -> Bus Creator3/2  "mu"
  Bus Creator/1 -> Bus Creator3/1  "z"
  Demux/2 -> Bus Creator/2  "G_FR_z"
  Demux/3 -> Bus Creator/3  "G_RL_z"
  Demux/1 -> Bus Creator/1  "G_FL_z"
  Demux/4 -> Bus Creator/4  "G_RR_z"
  Signal Specification/1 -> Demux/1
  Constant1/1 -> Signal Specification/1
  Demux1/2 -> Bus Creator2/2  "mu_FR"
  Demux1/1 -> Bus Creator2/1  "mu_FL"
  Demux1/3 -> Bus Creator2/3  "mu_RL"
  Demux1/4 -> Bus Creator2/4  "mu_RR"

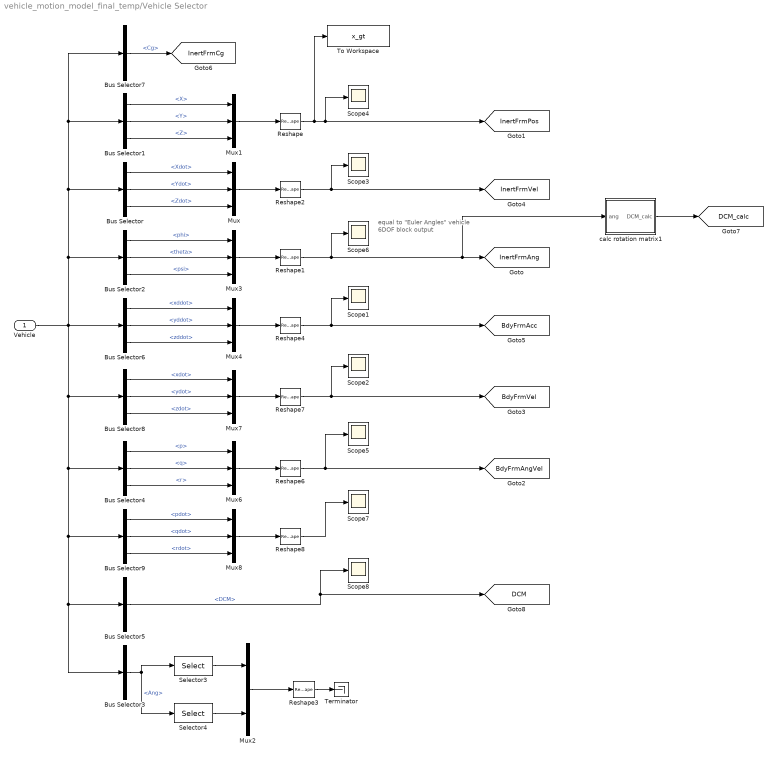
== system vehicle_motion_model_final_temp/Vehicle Selector ==
  note: equal to "Euler Angles" vehicle 6DOF block output
  Vehicle : Inport
  Bus Selector : BusSelector  OutputSignals=Vehicle.InertFrm.Cg.Vel.Xdot,Vehicle.InertFrm.Cg.Vel.Ydot,Vehicle.InertFrm.Cg.Vel.Zdot
  Bus Selector1 : BusSelector  OutputSignals=Vehicle.InertFrm.Cg.Disp.X,Vehicle.InertFrm.Cg.Disp.Y,Vehicle.InertFrm.Cg.Disp.Z
  Bus Selector2 : BusSelector  OutputSignals=Vehicle.InertFrm.Cg.Ang.phi,Vehicle.InertFrm.Cg.Ang.theta,Vehicle.InertFrm.Cg.Ang.psi
  Bus Selector3 : BusSelector  OutputSignals=Suspension.Whl.Ang
  Bus Selector4 : BusSelector  OutputSignals=Vehicle.BdyFrm.Cg.AngVel.p,Vehicle.BdyFrm.Cg.AngVel.q,Vehicle.BdyFrm.Cg.AngVel.r
  Bus Selector5 : BusSelector  OutputSignals=Vehicle.BdyFrm.Cg.DCM
  Bus Selector6 : BusSelector  OutputSignals=Vehicle.BdyFrm.Cg.Abe.xddot,Vehicle.BdyFrm.Cg.Abe.yddot,Vehicle.BdyFrm.Cg.Abe.zddot
  Bus Selector7 : BusSelector  OutputSignals=Vehicle.InertFrm.Cg
  Bus Selector8 : BusSelector  OutputSignals=Vehicle.BdyFrm.Cg.Vel.xdot,Vehicle.BdyFrm.Cg.Vel.ydot,Vehicle.BdyFrm.Cg.Vel.zdot
  Bus Selector9 : BusSelector  OutputSignals=Vehicle.BdyFrm.Cg.AngAcc.pdot,Vehicle.BdyFrm.Cg.AngAcc.qdot,Vehicle.BdyFrm.Cg.AngAcc.rdot
  Mux{,1,3..4,6..8} (7 alike) : Mux  Inputs=3
  Mux2 : Mux  Inputs=2
  Reshape{,1..4,6..8} (8 alike) : Reshape  OutputDimensionality=Column vector (2-D)
  Scope{1..8} (8 alike) : Scope
  Selector3 : Selector  NumberOfDimensions=2  InputPortWidth=6  IndexOptions=Index vector (dialog),Index vector (dialog)  Indices=3,[1 2]  OutputSizes=1,1
  Selector4 : Selector  NumberOfDimensions=2  InputPortWidth=6  IndexOptions=Index vector (dialog),Index vector (dialog)  Indices=3,[3 4]  OutputSizes=1,1
  Terminator : Terminator
  To Workspace : ToWorkspace  VariableName=x_gt  SaveFormat=Timeseries  SampleTime=-1
  calc rotation matrix1 : MATLAB Function  TreatAsAtomicUnit=on
  tag scope: BdyFrmAcc=global, BdyFrmAngVel=global, BdyFrmVel=global, DCM=global, DCM_calc=global, InertFrmAng=global, InertFrmCg=global, InertFrmPos=global, InertFrmVel=global
  wires:
  Mux2/1 -> Reshape3/1
  Mux/1 -> Reshape2/1
  Mux1/1 -> Reshape/1
  Bus Selector/1 -> Mux/1  "<Xdot>"
  Bus Selector1/1 -> Mux1/1  "<X>"
  Bus Selector1/2 -> Mux1/2  "<Y>"
  Bus Selector1/3 -> Mux1/3  "<Z>"
  Mux3/1 -> Reshape1/1
  Bus Selector2/3 -> Mux3/3  "<psi>"
  Bus Selector2/2 -> Mux3/2  "<theta>"
  Bus Selector2/1 -> Mux3/1  "<phi>"
  Selector3/1 -> Mux2/1
  Selector4/1 -> Mux2/2
  Bus Selector3/1 -> Selector3/1, Selector4/1  "<Ang>"
  Bus Selector6/1 -> Mux4/1  "<xddot>"
  Bus Selector6/2 -> Mux4/2  "<yddot>"
  Bus Selector6/3 -> Mux4/3  "<zddot>"
  Bus Selector4/1 -> Mux6/1  "<p>"
  Bus Selector4/2 -> Mux6/2  "<q>"
  Bus Selector4/3 -> Mux6/3  "<r>"
  Mux4/1 -> Reshape4/1
  Mux6/1 -> Reshape6/1
  Reshape3/1 -> Terminator/1
  Reshape/1 -> [InertFrmPos], Scope4/1, To Workspace/1
  Reshape1/1 -> calc rotation matrix1/1(ang), [InertFrmAng], Scope6/1
  Reshape4/1 -> [BdyFrmAcc], Scope1/1
  Bus Selector9/1 -> Mux8/1  "<pdot>"
  Bus Selector9/2 -> Mux8/2  "<qdot>"
  Bus Selector9/3 -> Mux8/3  "<rdot>"
  Mux8/1 -> Reshape8/1
  Bus Selector8/1 -> Mux7/1  "<xdot>"
  Bus Selector8/2 -> Mux7/2  "<ydot>"
  Bus Selector8/3 -> Mux7/3  "<zdot>"
  Mux7/1 -> Reshape7/1
  Reshape2/1 -> [InertFrmVel], Scope3/1
  Bus Selector/2 -> Mux/2  "<Ydot>"
  Bus Selector/3 -> Mux/3  "<Zdot>"
  Bus Selector7/1 -> [InertFrmCg]  "<Cg>"
  Bus Selector5/1 -> [DCM], Scope8/1  "<DCM>"
  Reshape7/1 -> [BdyFrmVel], Scope2/1
  Reshape6/1 -> [BdyFrmAngVel], Scope5/1
  Reshape8/1 -> Scope7/1
  calc rotation matrix1/1(DCM_calc) -> [DCM_calc]
  Vehicle/1 -> Bus Selector6/1, Bus Selector2/1, Bus Selector/1, Bus Selector1/1, Bus Selector7/1, Bus Selector8/1, Bus Selector4/1, Bus Selector9/1, Bus Selector5/1, Bus Selector3/1

== system vehicle_motion_model_final_temp/BINS/Subsystem ==
  True : Inport
  BINS : Inport  Port=2
  Scope1 : Scope  NumInputPorts=3
  Sum2 : Sum  Inputs=+-|
  wires:
  True/1 -> Sum2/1, Scope1/1
  BINS/1 -> Scope1/2, Sum2/2
  Sum2/1 -> Scope1/3

== system vehicle_motion_model_final_temp/BINS/Subsystem1 ==
  True : Inport
  BINS : Inport  Port=2
  Scope1 : Scope  NumInputPorts=3
  Sum2 : Sum  Inputs=+-|
  wires:
  True/1 -> Sum2/1, Scope1/1
  BINS/1 -> Scope1/2, Sum2/2
  Sum2/1 -> Scope1/3

== system vehicle_motion_model_final_temp/BINS/Three-axis Inertial Measurement Unit2 ==
  A_b : Inport  Unit=m/s^2  PortDimensions=3
  w : Inport  Port=2  Unit=rad/s  PortDimensions=3
  w_dot : Inport  Port=3  Unit=rad/s^2  PortDimensions=3
  CG : Inport  Port=4  Unit=m  PortDimensions=3
  g : Inport  Port=5  Unit=m/s^2  PortDimensions=3
  Acceleration Conversion : Subsystem
  Disallow CGS : UnitConfiguration  UnitSystemsStr=English,SI,SI (extended)  AllowAllUnitSystems=off
  Three-axis Accelerometer : Subsystem  AncestorBlock=aerolibnav/Three-axis Accelerometer  mask(Three-axis Accelerometer){units=Metric (MKS), acc=imu, gtype=on, dtype_a=off, w_a=w_a, z_a=z_a, a_sf_cc=a_sf_cc, a_bias=a_bias, a_Ts=i_Ts, a_rand=on, a_seeds=i_seeds(1:3), a_pow=i_pow(1:3), a_sat=a_sat}
      mask prompts: units "aeroblks:aeroblknav:blockThreeaxisAccelerometerParamUnits"; acc "aeroblks:aeroblknav:blockThreeaxisAccelerometerParamAccelerometerlocation"; gtype "aeroblks:aeroblknav:blockThreeaxisAccelerometerParamSubtractgravity"; dtype_a "aeroblks:aeroblknav:blockThreeaxisAccelerometerParamSecondorderdynamics"; w_a "aeroblks:aeroblknav:blockThreeaxisAccelerometerParamNaturalfrequencyradsec"; z_a "aeroblks:aeroblknav:blockThreeaxisAccelerometerParamDampingratio"; a_sf_cc "aeroblks:aeroblknav:blockThreeaxisAccelerometerParamScalefactorsandcrosscoupling"; a_bias "aeroblks:aeroblknav:blockThreeaxisAccelerometerParamMeasurementbias"; a_Ts "aeroblks:aeroblknav:blockThreeaxisAccelerometerParamUpdateratesec"; a_rand "aeroblks:aeroblknav:blockThreeaxisAccelerometerParamNoiseon"; a_seeds "aeroblks:aeroblknav:blockThreeaxisAccelerometerParamNoiseseeds"; a_pow "aeroblks:aeroblknav:blockThreeaxisAccelerometerParamNoisepower"; a_sat "aeroblks:aeroblknav:blockThreeaxisAccelerometerParamLowerandupperoutputlimits"
      mask help: aeroblks:aeroblknav:blockThreeaxisAccelerometerDesc
      mask init:
      | par = a_Ts;
      | block = gcb;
      | ports=aeroicon('aeroblkaccel','icon',par);
      | a_satl = a_sat(1:3);
      | a_sath = a_sat(4:6);
      mask Help: eval('asbhelp');
      mask TypeOptions units: aeroblks:aeroblknav:blockThreeaxisAccelerometerParamComboMetricMKS | aeroblks:aeroblknav:blockThreeaxisAccelerometerParamComboEnglish
      mask Callback gtype: aeroicon('aeroblkaccel')
      mask Callback dtype_a: aeroicon('aeroblkaccel')
      mask Callback a_rand: aeroicon('aeroblkaccel')
      mask DialogControl ParameterTabVar0 Prompt: Main
      mask DialogControl units Prompt: Units:
      mask DialogControl acc Prompt: Accelerometer location:
      mask DialogControl gtype Prompt: Subtract gravity:
      mask DialogControl dtype_a Prompt: Second-order dynamics
      mask DialogControl w_a Prompt: Natural frequency (rad/sec):
      mask DialogControl z_a Prompt: Damping ratio:
      mask DialogControl a_sf_cc Prompt: Scale factors and cross-coupling:
      mask DialogControl a_bias Prompt: Measurement bias:
      mask DialogControl a_Ts Prompt: Update rate (sec):
      mask DialogControl ParameterTabVar01 Prompt: Noise
      mask DialogControl a_rand Prompt: Noise on
      mask DialogControl a_seeds Prompt: Noise seeds:
      mask DialogControl a_pow Prompt: Noise power:
      mask DialogControl a_sat Prompt: Lower and upper output limits:
      mask Display:
      | port_label(ports(1).type,ports(1).port,ports(1).txt,'texmode','on');
      | port_label(ports(2).type,ports(2).port,ports(2).txt,'texmode','on');
      | port_label(ports(3).type,ports(3).port,ports(3).txt,'texmode','on');
      | port_label(ports(4).type,ports(4).port,ports(4).txt,'texmode','on');
      | port_label(ports(5).type,ports(5).port,ports(5).txt,'texmode','on');
      | port_label(ports(6).type,ports(6).port,ports(6).txt,'texmode','on');
  Three-axis Gyroscope : Subsystem  AncestorBlock=aerolibnav/Three-axis Gyroscope  mask(Three-axis Gyroscope){dtype_g=off, w_g=w_g, z_g=z_g, g_sf_cc=g_sf_cc, g_bias=g_bias, g_sen=g_sens, g_Ts=i_Ts, g_rand=on, g_seeds=i_seeds(4:6), g_pow=i_pow(4:6), g_sat=g_sat}
      mask prompts: dtype_g "aeroblks:aeroblknav:blockThreeaxisGyroscopeParamSecondorderdynamics"; w_g "aeroblks:aeroblknav:blockThreeaxisGyroscopeParamNaturalfrequencyradsec"; z_g "aeroblks:aeroblknav:blockThreeaxisGyroscopeParamDampingratio"; g_sf_cc "aeroblks:aeroblknav:blockThreeaxisGyroscopeParamScalefactorsandcrosscoupling"; g_bias "aeroblks:aeroblknav:blockThreeaxisGyroscopeParamMeasurementbias"; g_sen "aeroblks:aeroblknav:blockThreeaxisGyroscopeParamGsensitivebias"; g_Ts "aeroblks:aeroblknav:blockThreeaxisGyroscopeParamUpdateratesec"; g_rand "aeroblks:aeroblknav:blockThreeaxisGyroscopeParamNoiseon"; g_seeds "aeroblks:aeroblknav:blockThreeaxisGyroscopeParamNoiseseeds"; g_pow "aeroblks:aeroblknav:blockThreeaxisGyroscopeParamNoisepower"; g_sat "aeroblks:aeroblknav:blockThreeaxisGyroscopeParamLowerandupperoutputlimits"
      mask help: aeroblks:aeroblknav:blockThreeaxisGyroscopeDesc
      mask init:
      | par = g_Ts;
      | block = gcb;
      | g_satl = g_sat(1:3);
      | g_sath = g_sat(4:6);
      | ports=aeroicon('aeroblkgyro','icon',par);
      mask Help: eval('asbhelp');
      mask Callback dtype_g: aeroicon('aeroblkgyro');
      mask Callback g_rand: aeroicon('aeroblkgyro');
      mask DialogControl ParameterTabVar0 Prompt: Main
      mask DialogControl dtype_g Prompt: Second-order dynamics
      mask DialogControl w_g Prompt: Natural frequency (rad/sec):
      mask DialogControl z_g Prompt: Damping ratio:
      mask DialogControl g_sf_cc Prompt: Scale factors and cross-coupling:
      mask DialogControl g_bias Prompt: Measurement bias:
      mask DialogControl g_sen Prompt: G-sensitive bias:
      mask DialogControl g_Ts Prompt: Update rate (sec):
      mask DialogControl ParameterTabVar01 Prompt: Noise
      mask DialogControl g_rand Prompt: Noise on
      mask DialogControl g_seeds Prompt: Noise seeds:
      mask DialogControl g_pow Prompt: Noise power:
      mask DialogControl g_sat Prompt: Lower and upper output limits:
      mask Display:
      | port_label(ports(1).type,ports(1).port,ports(1).txt,'texmode','on');
      | port_label(ports(2).type,ports(2).port,ports(2).txt,'texmode','on');
      | port_label(ports(3).type,ports(3).port,ports(3).txt,'texmode','on');
  A_meas : Outport  Unit=m/s^2  VectorParamsAs1DForOutWhenUnconnected=off
  w_meas : Outport  Port=2  Unit=rad/s  VectorParamsAs1DForOutWhenUnconnected=off
  wires:
  g/1 -> Three-axis Accelerometer/5(g)
  Acceleration Conversion/1(inherit) -> Three-axis Gyroscope/2(G's)
  w_dot/1 -> Three-axis Accelerometer/3(pdot qdot rdot)
  CG/1 -> Three-axis Accelerometer/4(CG)
  w/1 -> Three-axis Accelerometer/2(p q r), Three-axis Gyroscope/1(p q r)
  A_b/1 -> Three-axis Accelerometer/1(Ab), Acceleration Conversion/1(acceleration)
  Three-axis Gyroscope/1((p q r)_meas) -> w_meas/1
  Three-axis Accelerometer/1(Ameas) -> A_meas/1
